simulink library "asbCubeSatActuatorsLib"  (R2026a)
settings: Solver=VariableStepAuto
libraries: $bdroot x1
settings Model: Creator=The MathWorks, Inc.  LastModifiedBy=The MathWorks, Inc.

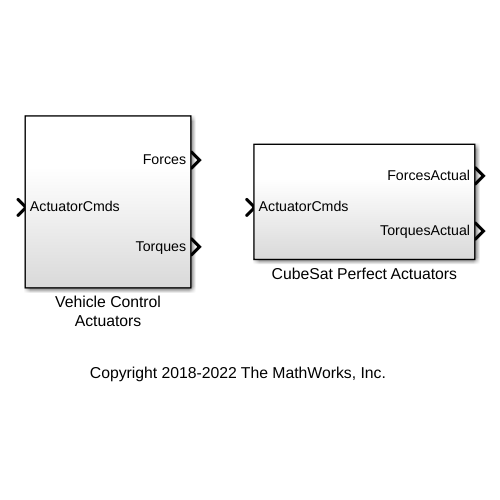
[thumbnail: Simulink's stored preview of the top-level diagram]
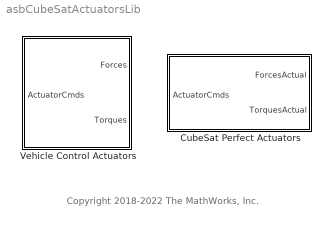
== system asbCubeSatActuatorsLib ==
  note: Copyright 2018-2022 The MathWorks, Inc.
  CubeSat Perfect Actuators : Subsystem
  Vehicle Control Actuators : Subsystem  RequirementInfo={} %GIDa_fba6ccff_ebba_4f2b_aabb_40150f996586

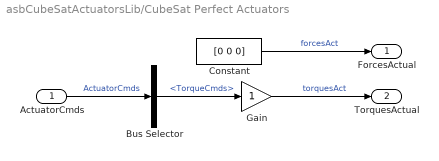
== system asbCubeSatActuatorsLib/CubeSat Perfect Actuators ==
  ActuatorCmds : Inport  OutDataTypeStr=Bus: FCSOutBus
  Bus Selector : BusSelector  OutputSignals=ACSOut.TorqueCmds
  Constant : Constant  Value=[0 0 0]
  Gain : Gain
  ForcesActual : Outport  VectorParamsAs1DForOutWhenUnconnected=off
  TorquesActual : Outport  Port=2  VectorParamsAs1DForOutWhenUnconnected=off
  wires:
  ActuatorCmds/1 -> Bus Selector/1  "ActuatorCmds"
  Bus Selector/1 -> Gain/1  "<TorqueCmds>"
  Gain/1 -> TorquesActual/1  "torquesAct"
  Constant/1 -> ForcesActual/1  "forcesAct"

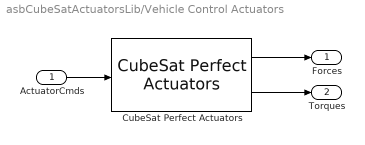
== system asbCubeSatActuatorsLib/Vehicle Control Actuators ==
  ActuatorCmds : Inport  RequirementInfo={} %GIDa_020f38c4_9e26_4002_9065_5d46819fcfcb
  CubeSat Perfect Actuators : $bdroot/CubeSat Perfect Actuators  SystemSampleTime=-1  VariantActivationTime=update diagram  EmptyChoice=off  PassThrough=off  PassThroughVariantControl=(default)  EmptyChoiceVariantControl=(default)  AllowFlexibleInterface=on  Latency=0  AutoFrameSizeCalculation=off
  " Forces" : Outport  RequirementInfo={} %GIDa_e46e2c30_d205_4036_910c_a099c6c54d17  VectorParamsAs1DForOutWhenUnconnected=off
  " Torques" : Outport  RequirementInfo={} %GIDa_67b5453a_f72e_4aa8_be3c_a57a924d68da  Port=2  VectorParamsAs1DForOutWhenUnconnected=off
  wires:
  ActuatorCmds/1 -> CubeSat Perfect Actuators/1
  CubeSat Perfect Actuators/2 -> " Torques"/1
  CubeSat Perfect Actuators/1 -> " Forces"/1
